simulink model "TASARIM"  (R2024a)
settings: Solver=VariableStepAuto  StartTime=0.0  StopTime=5  RelTol=1e-3
values from neighbouring files (symbols this model uses):
  B = 0.02    [PID_projesi_son_hal.m]
  dz = cell2mat(dz)    [PID_projesi_son_hal.m]
  j = 0.072    [PID_projesi_son_hal.m]
  K_i = 1.24    [PID_projesi_son_hal.m]
  Kb = 1.24    [PID_projesi_son_hal.m]
  Kd = (z1/sin(beta))*(((Ki*sin(beta))/(z1-2*cos(beta)+(1/z1)))+(sin(fi)/Gp_z1))    [PID_projesi_son_hal.m]
  Ki = Kv*T/limit    [PID_projesi_son_hal.m]
  Kp = (-cos(fi)/Gp_z1)-(2*Ki*z1*((z1-cos(beta))/(z1^2-2*z1*cos(beta)+1)))+((-z1*sin(fi)+cos(beta)*sin(fi))/(Gp_z1*sin(beta)))    [PID_projesi_son_hal.m]
  La = 1.4    [PID_projesi_son_hal.m]
  nz = cell2mat(nz)    [PID_projesi_son_hal.m]
  R = 2.8    [PID_projesi_son_hal.m]
  Ref = 24    [PID_projesi_son_hal.m]
  Ref_max = 24    [PID_projesi_son_hal.m]
  Ref_min = 24    [PID_projesi_son_hal.m]
  T = 10e-3    (= 0.01)    [PID_projesi_son_hal.m]
  Ts = T    [PID_projesi_son_hal.m]
libraries: spsIGBTDiodeLib x16, simulink_extras x11, simulink x8, spsDCMachineLib x4, spsDCVoltageSourceLib x4, spsGroundLib x4, spsVoltageMeasurementLib x4, sps_lib x1
settings Model: Creator=ESMA  LastModifiedBy=ESMA

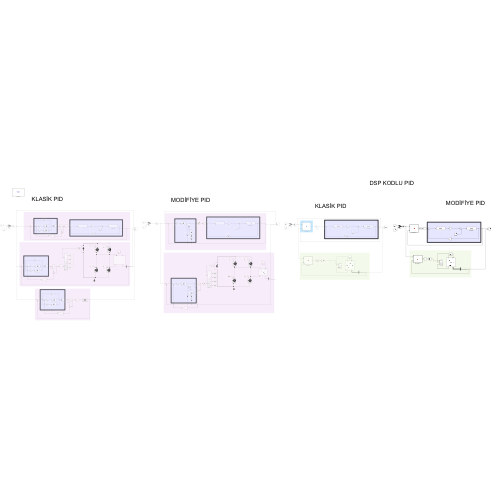
[thumbnail: Simulink's stored preview of the top-level diagram]
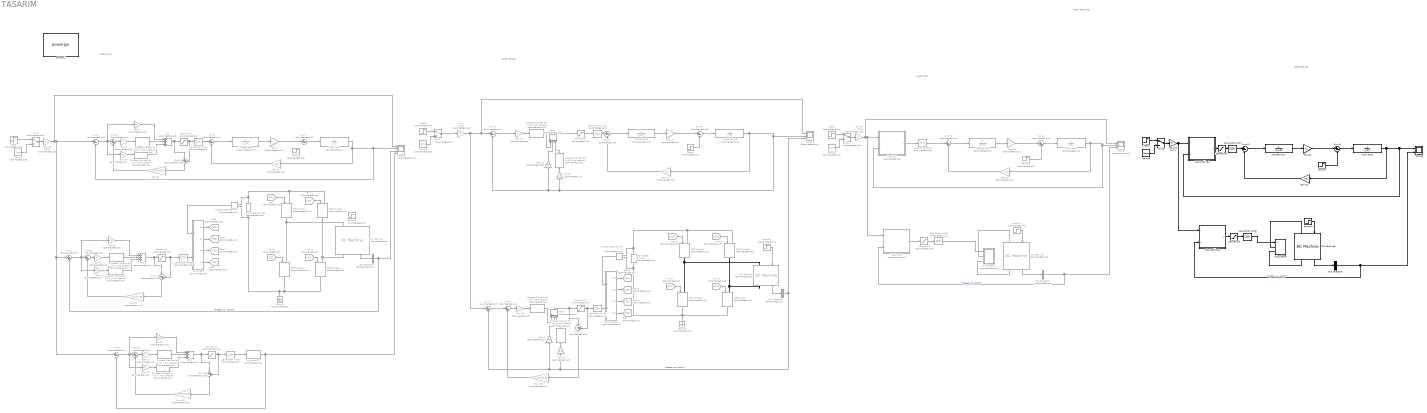
== system TASARIM ==
  note: KLASİK PID
  note: KLASİK PID
  note: MODİFİYE PID
  note: DSP KODLU PID
  note: MODİFİYE PID
  Add : Sum  Commented=on  Inputs=+++
  Add1 : Sum  Commented=on  Inputs=+--
  Add2 : Sum  Commented=on  Inputs=+++
  Add3 : Sum  Commented=on  Inputs=+--
  Add4 : Sum  Commented=on  Inputs=+++
  Bus Selector1 : BusSelector  Commented=on  OutputSignals=Speed wm (rad/s)
  Bus Selector2 : BusSelector  Commented=on  OutputSignals=Speed wm (rad/s)
  Bus Selector3 : BusSelector  OutputSignals=Speed wm (rad/s)
  Bus Selector4 : BusSelector  Commented=on  OutputSignals=Speed wm (rad/s)
  DC Machine : spsDCMachineLib/DC Machine  Commented=on  PresetModel=No  MechanicalLoad=Torque TL  FieldType=Permanent magnet  ShowDetailedParameters=on  MeasurementBus=off  RLa=[R La ]  RLf="[ 240  120]"  Laf=1.8  MachineConstant=Back-emf constant (V/rpm)  Ke=Kb*(2*pi)/60  Kt=1.8  J=j  Bm=B  Tf=0  w0=0  Ifinit=1  TsPowergui=0  TsBlock=-1
  DC Machine1 : spsDCMachineLib/DC Machine  Commented=on  PresetModel=No  MechanicalLoad=Torque TL  FieldType=Permanent magnet  ShowDetailedParameters=on  MeasurementBus=off  RLa=[R La ]  RLf="[ 240  120]"  Laf=1.8  MachineConstant=Back-emf constant (V/rpm)  Ke=Kb*(2*pi)/60  Kt=1.8  J=j  Bm=B  Tf=0  w0=0  Ifinit=1  TsPowergui=0  TsBlock=-1
  DC Machine2 : spsDCMachineLib/DC Machine  Commented=on  PresetModel=No  MechanicalLoad=Torque TL  FieldType=Permanent magnet  ShowDetailedParameters=on  MeasurementBus=off  RLa=[R La ]  RLf="[ 240  120]"  Laf=1.8  MachineConstant=Back-emf constant (V/rpm)  Ke=Kb*(2*pi)/60  Kt=1.8  J=j  Bm=B  Tf=0  w0=0  Ifinit=1  TsPowergui=0  TsBlock=-1
  DC Machine3 : spsDCMachineLib/DC Machine  PresetModel=No  MechanicalLoad=Torque TL  FieldType=Permanent magnet  ShowDetailedParameters=on  MeasurementBus=off  RLa=[R La ]  RLf="[ 240  120]"  Laf=1.8  MachineConstant=Back-emf constant (V/rpm)  Ke=Kb*(2*pi)/60  Kt=1.8  J=j  Bm=B  Tf=0  w0=0  Ifinit=1  TsPowergui=0  TsBlock=-1
  DC Voltage Source : spsDCVoltageSourceLib/DC Voltage Source  Commented=on  Amplitude=24  Measurements=None
  DC Voltage Source1 : spsDCVoltageSourceLib/DC Voltage Source  Commented=on  Amplitude=24  Measurements=None
  Discrete Transfer Fcn (with initial states){1..2,5,7,9} (5 alike) : simulink_extras/Additional Discrete/Discrete Transfer Fcn (with initial states)  Commented=on  N=[1 0]  D=[1 -1]  X0=[1]  TS=T
  Discrete Transfer Fcn (with initial states){3..4,6,8,10} (5 alike) : simulink_extras/Additional Discrete/Discrete Transfer Fcn (with initial states)  Commented=on  N=[1 -1]  D=[1 0]  X0=[1]  TS=T
  From : From  Commented=on  GotoTag=G1
  From1 : From  Commented=on  GotoTag=G3
  From2 : From  Commented=on  GotoTag=G4
  From3 : From  Commented=on  GotoTag=G2
  From4 : From  Commented=on  GotoTag=G11
  From5 : From  Commented=on  GotoTag=G31
  From6 : From  Commented=on  GotoTag=G41
  From7 : From  Commented=on  GotoTag=G21
  Gain{1,6,10,16..17} (5 alike) : Gain  Commented=on  Gain=Kd
  Gain11 : Gain  Commented=on  Gain=K_i
  Gain12 : Gain  Commented=on  Gain=Kb
  Gain{4,7..8,13,27} (5 alike) : Gain  Commented=on  Gain=Kp
  Gain{5,9,14..15,33} (5 alike) : Gain  Commented=on  Gain=Ki
  Gain{18,26,31..32} (4 alike) : Gain  Commented=on  Gain=Ki/Kd*4.35
  Gain19 : Gain  Commented=on  Gain=K_i
  Gain2 : Gain  Commented=on  Gain=K_i
  Gain20 : Gain  Commented=on  Gain=Kb
  Gain21 : Gain  Gain=K_i
  Gain22 : Gain  Gain=Kb
  Gain24 : Gain  Commented=on  Gain=18/24
  Gain25 : Gain  Gain=18/24
  Gain28 : Gain  Commented=on  Gain=18/24
  Gain3 : Gain  Commented=on  Gain=Kb
  Giriş : ManualSwitch  Commented=on
  Giriş1 : ManualSwitch  Commented=on
  Giriş2 : ManualSwitch  Commented=on
  Giriş3 : ManualSwitch
  Goto : Goto  Commented=on  GotoTag=G1
  Goto1 : Goto  Commented=on  GotoTag=G2
  Goto2 : Goto  Commented=on  GotoTag=G3
  Goto3 : Goto  Commented=on  GotoTag=G4
  Goto4 : Goto  Commented=on  GotoTag=G11
  Goto5 : Goto  Commented=on  GotoTag=G21
  Goto6 : Goto  Commented=on  GotoTag=G31
  Goto7 : Goto  Commented=on  GotoTag=G41
  Ground : spsGroundLib/Ground  Commented=on  LConnTagsString=a
  Ground1 : spsGroundLib/Ground  Commented=on  LConnTagsString=a
  IGBT/Diode{,1..7} (8 alike) : spsIGBTDiodeLib/IGBT//Diode  Commented=on  Ron=1e-6  Rs=1e5  Cs=inf  Measurements=off
  Klasik PID : MATLAB Function  Commented=on  TreatAsAtomicUnit=on
  Klasik PID1 : MATLAB Function  Commented=on  TreatAsAtomicUnit=on
  PID_Modifiye1 : MATLAB Function  TreatAsAtomicUnit=on
  PID_Modifiye2 : MATLAB Function  TreatAsAtomicUnit=on
  Ramp1 : simulink/Sources/Ramp  Commented=on  slope=Ref  start=0  InitialOutput=0
  Ramp2 : simulink/Sources/Ramp  Commented=on  slope=Ref  start=0  InitialOutput=0
  Ramp3 : simulink/Sources/Ramp  slope=Ref  start=0  InitialOutput=0
  Ramp4 : simulink/Sources/Ramp  Commented=on  slope=Ref  start=0  InitialOutput=0
  Saturation{1,3..4,7..9} (6 alike) : Saturate  Commented=on  UpperLimit=Ref  LowerLimit=-Ref
  Saturation5 : Saturate  UpperLimit=Ref  LowerLimit=-Ref
  Saturation6 : Saturate  UpperLimit=Ref  LowerLimit=-Ref
  Scope : Scope  Commented=on  NumInputPorts=3
  Scope1 : Scope  NumInputPorts=2
  Scope3 : Scope  Commented=on  NumInputPorts=3
  Scope4 : Scope  Commented=on  NumInputPorts=4
  Step1 : Step  Commented=on  Time=0  After=Ref  SampleTime=0
  Step2 : Step  Commented=on  Time=0  After=Ref  SampleTime=0
  Step3 : Step  Commented=on  Time=0  After=Ref  SampleTime=0
  Step4 : Step  Time=0  After=Ref  SampleTime=0
  Step5 : Step  Commented=on  Time=0  After=0  SampleTime=0
  Subsystem : Subsystem  Commented=on
  Subsystem1 : Subsystem  Commented=on
  Subsystem2 : Subsystem
  Subsystem3 : Subsystem  Commented=on
  Sum{1..5,7..9,11,13..14} (11 alike) : Sum  Commented=on  Inputs=|+-
  Sum{12,17,19,21} (4 alike) : Sum  Commented=on  Inputs=|-+
  Sum15 : Sum  Inputs=|+-
  Sum16 : Sum  Inputs=|+-
  Sum{6,18,20,22} (4 alike) : Sum  Commented=on  Inputs=|++
  Transfer Fcn1 : TransferFcn  Commented=on  Denominator=[La R]
  Transfer Fcn2 : TransferFcn  Denominator=[La R]
  Transfer Fcn3 : TransferFcn  Commented=on  Denominator=[La R]
  Transfer Fcn6 : TransferFcn  Commented=on  Denominator=[La R]
  Voltage Measurement : spsVoltageMeasurementLib/Voltage Measurement  Commented=on  PhasorSimulation=off  OutputType=Complex  PSBequivalent=0
  Voltage Measurement1 : spsVoltageMeasurementLib/Voltage Measurement  Commented=on  PhasorSimulation=off  OutputType=Complex  PSBequivalent=0
  Zero-Order Hold{1..6,9} (7 alike) : ZeroOrderHold  Commented=on  SampleTime=T
  Zero-Order Hold7 : ZeroOrderHold  SampleTime=T
  Zero-Order Hold8 : ZeroOrderHold  SampleTime=T
  bozucu{,1..3,5} (5 alike) : Step  Commented=on  Time=0  After=0  SampleTime=0
  bozucu4 : Step  Time=0  After=0  SampleTime=0
  bozucu6 : Step  Time=0  After=0  SampleTime=0
  giriş : Gain  Commented=on  Gain=18/24
  klasik PID : TransferFcn  Commented=on  Denominator=[j B]
  klasik PID1 : TransferFcn  Commented=on  Denominator=[j B]
  klasik PID2 : TransferFcn  Denominator=[j B]
  modifiyeli PID : TransferFcn  Commented=on  Denominator=[j B]
  powergui : sps_lib/powergui  Priority=1  SimulationMode=Discrete  SampleTime=1e-6  frequency=60  Iterations=50  frequencyindice=0  Pbase=100e6  ErrMax=1e-4  UnitsV=kV  UnitsW=MW  buscounter=0  FunctionMessages=off  echomessages=off  EnableUseOfTLC=off  CurrentSourceSwitches=off  DisableSnubberDevices=off  DisableRonSwitches=off  DisableVfSwitches=off  DisplayEquations=off  AutomaticDiscreteSolvers=off  SolverType=Tustin/Backward Euler (TBE)  Interpol=off  ExternalGateDelay=off  methode=off  Ts=100  x0status=blocks  SPID=on  SwTol=0  HookPort=off  NonlinearTolerance=1e-4  nMaxIteration=100  ContinueOnMaxIteration=off  RestoreLinks=warning  ResistiveCurrentMeasurement=off  Frange=[0:2:500]  Ylog=off  Xlog=on  ShowGrid=off  save=off  variable=ZData  structure=0  ZoomFFT=off  StartTime=0.0  cycles=1  DisplayStyle=1  fundamental=60  FreqAxis=off  MaxFrequency=1000  frequencyindicesteady=1  RmsSteady=1  display=off
  z_domeniTF : simulink_extras/Additional Discrete/Discrete Transfer Fcn (with initial states)  Commented=on  N=[nz]  D=[dz]  X0=[0]  TS=T
  wires:
  klasik PID/1 -> Gain3/1, Scope4/2, Sum2/2
  Gain7/1 -> Add/1
  Gain9/1 -> Discrete Transfer Fcn (with initial states)2/1
  Step2/1 -> Giriş/1
  Sum3/1 -> Transfer Fcn6/1
  Discrete Transfer Fcn (with initial states)3/1 -> Add/3
  Sum2/1 -> Gain7/1, Gain10/1, Sum20/1
  Sum7/1 -> klasik PID/1
  Gain10/1 -> Discrete Transfer Fcn (with initial states)3/1
  Transfer Fcn6/1 -> Gain2/1
  Ramp1/1 -> Giriş/2
  Gain2/1 -> Sum7/1
  Discrete Transfer Fcn (with initial states)2/1 -> Add/2
  Gain3/1 -> Sum3/2
  Discrete Transfer Fcn (with initial states)5/1 -> Add2/2
  Gain1/1 -> Discrete Transfer Fcn (with initial states)6/1
  Discrete Transfer Fcn (with initial states)6/1 -> Add2/3
  Gain4/1 -> Add2/1
  Gain5/1 -> Discrete Transfer Fcn (with initial states)5/1
  Sum1/1 -> Sum18/1, Gain1/1, Gain4/1
  Zero-Order Hold1/1 -> Sum3/1
  Sum11/1 -> modifiyeli PID/1
  Zero-Order Hold6/1 -> Subsystem3/1(uconT)
  bozucu5/1 -> DC Machine2/1
  DC Machine2/1 -> Bus Selector2/1
  Saturation1/1 -> Zero-Order Hold5/1, Sum12/2
  PID_Modifiye2/1(u) -> Saturation6/1
  Zero-Order Hold8/1 -> Subsystem2/1(uconT)
  Ramp2/1 -> Giriş2/2
  Gain8/1 -> Add3/2
  Gain22/1 -> Sum15/2
  Saturation6/1 -> Zero-Order Hold8/1
  Gain16/1 -> Discrete Transfer Fcn (with initial states)8/1
  bozucu2/1 -> DC Machine1/1
  Gain11/1 -> Sum11/1
  Subsystem1/1(G1) -> Goto4/1
  Gain15/1 -> Discrete Transfer Fcn (with initial states)7/1
  Step5/1 -> Sum11/2
  Zero-Order Hold5/1 -> Subsystem1/2(uconT)
  bozucu3/1 -> Sum14/2
  Zero-Order Hold4/1 -> Sum13/1
  Subsystem1/2(G2) -> Goto5/1
  Transfer Fcn1/1 -> Gain19/1
  Sum12/1 -> Gain18/1
  Subsystem1/4(G4) -> Goto7/1
  Gain14/1 -> Discrete Transfer Fcn (with initial states)1/1
  Sum4/1 -> Sum6/1
  Discrete Transfer Fcn (with initial states)8/1 -> Add3/3
  Gain25/1 -> PID_Modifiye2/1(r), PID_Modifiye1/1(r)
  Discrete Transfer Fcn (with initial states)1/1 -> Add1/1
  Ramp3/1 -> Giriş3/2
  PID_Modifiye1/1(u) -> Saturation5/1
  Transfer Fcn3/1 -> Gain11/1
  Discrete Transfer Fcn (with initial states)7/1 -> Add3/1
  Saturation3/1 -> Zero-Order Hold6/1
  Gain19/1 -> Sum14/1
  Sum16/1 -> klasik PID2/1
  Sum15/1 -> Transfer Fcn2/1
  Discrete Transfer Fcn (with initial states)4/1 -> Add1/3
  DC Machine1/1 -> Bus Selector1/1
  Gain6/1 -> Discrete Transfer Fcn (with initial states)4/1
  klasik PID2/1 -> Scope1/1, PID_Modifiye1/2(c), Gain22/1
  From5/1 -> IGBT/Diode5/1
  Zero-Order Hold2/1 -> Sum9/1
  Gain21/1 -> Sum16/1
  Zero-Order Hold7/1 -> Sum15/1
  Sum9/1 -> Transfer Fcn3/1
  Sum13/1 -> Transfer Fcn1/1
  Saturation5/1 -> Zero-Order Hold7/1
  Giriş1/1 -> giriş/1
  bozucu4/1 -> Sum16/2
  Step4/1 -> Giriş3/1
  Gain20/1 -> Sum13/2
  DC Machine3/1 -> Bus Selector3/1
  Transfer Fcn2/1 -> Gain21/1
  Gain18/1 -> Sum6/2
  Gain12/1 -> Sum9/2
  Subsystem1/3(G3) -> Goto6/1
  klasik PID1/1 -> Gain20/1, Scope/2, Klasik PID/2(c)
  Klasik PID1/1(u) -> Saturation3/1
  From6/1 -> IGBT/Diode7/1
  Step3/1 -> Giriş1/1
  From7/1 -> IGBT/Diode6/1
  From4/1 -> IGBT/Diode4/1
  Ramp4/1 -> Giriş1/2
  Step1/1 -> Giriş2/1
  Sum14/1 -> klasik PID1/1
  Gain13/1 -> Add1/2
  Klasik PID/1(u) -> Zero-Order Hold4/1
  Add1/1 -> Saturation4/1
  modifiyeli PID/1 -> Gain12/1, Gain6/1, Sum8/2, Gain13/1, Scope3/2
  Add3/1 -> Sum12/1, Saturation1/1
  Voltage Measurement1/1 -> Subsystem1/1(E)
  Sum8/1 -> Gain14/1
  Giriş2/1 -> Gain24/1
  bozucu6/1 -> DC Machine3/1
  Giriş3/1 -> Gain25/1
  giriş/1 -> Scope3/1, Sum8/1, Sum4/1
  Zero-Order Hold3/1 -> Subsystem/2(uconT)
  Voltage Measurement/1 -> Subsystem/1(E)
  From3/1 -> IGBT/Diode2/1
  Subsystem/1(G1) -> Goto/1
  From/1 -> IGBT/Diode/1
  Subsystem/2(G2) -> Goto1/1
  Subsystem/3(G3) -> Goto2/1
  From2/1 -> IGBT/Diode3/1
  DC Machine/1 -> Bus Selector4/1
  From1/1 -> IGBT/Diode1/1
  Subsystem/4(G4) -> Goto3/1
  Saturation4/1 -> Zero-Order Hold2/1
  z_domeniTF/1 -> Scope4/4, Sum5/2
  Add2/1 -> Saturation8/1, Sum17/1
  Gain31/1 -> Sum18/2
  Sum17/1 -> Gain31/1
  Sum18/1 -> Gain5/1
  Sum19/1 -> Gain32/1
  Add/1 -> Saturation7/1, Sum19/1
  Gain32/1 -> Sum20/2
  Sum20/1 -> Gain9/1
  Add4/1 -> Sum21/1, Saturation9/1
  Sum22/1 -> Gain33/1
  Sum5/1 -> Sum22/1, Gain17/1, Gain27/1
  Gain33/1 -> Discrete Transfer Fcn (with initial states)9/1
  Gain17/1 -> Discrete Transfer Fcn (with initial states)10/1
  Discrete Transfer Fcn (with initial states)9/1 -> Add4/2
  Discrete Transfer Fcn (with initial states)10/1 -> Add4/3
  Sum21/1 -> Gain26/1
  Gain26/1 -> Sum22/2
  Saturation9/1 -> Zero-Order Hold9/1, Sum21/2
  Gain27/1 -> Add4/1
  Zero-Order Hold9/1 -> z_domeniTF/1
  Bus Selector4/1 -> Scope4/3, Sum1/2  "<Speed wm (rad/s)>"
  Bus Selector1/1 -> Scope3/3, Gain16/1, Gain8/1, Sum4/2  "<Speed wm (rad/s)>"
  Sum6/1 -> Gain15/1
  Bus Selector3/1 -> Scope1/2, PID_Modifiye2/2(c)  "<Speed wm (rad/s)>"
  Bus Selector2/1 -> Scope/3, Klasik PID1/2(c)  "<Speed wm (rad/s)>"
  Saturation7/1 -> Sum19/2, Zero-Order Hold1/1
  Saturation8/1 -> Zero-Order Hold3/1, Sum17/2
  Giriş/1 -> Gain28/1
  Gain28/1 -> Scope4/1, Sum2/1, Sum1/1, Sum5/1
  Gain24/1 -> Scope/1, Klasik PID1/1(r), Klasik PID/1(r)
  connections:
  DC Machine1/RConn1 -- IGBT/Diode7/LConn1 -- IGBT/Diode5/RConn1
  Subsystem3/LConn1 -- DC Machine2/LConn1
  Subsystem3/LConn2 -- DC Machine2/RConn1
  Subsystem2/LConn1 -- DC Machine3/LConn1
  Subsystem2/LConn2 -- DC Machine3/RConn1
  Voltage Measurement1/LConn2 -- DC Voltage Source1/LConn1 -- IGBT/Diode7/RConn1 -- IGBT/Diode6/RConn1 -- Ground1/LConn1
  DC Voltage Source1/RConn1 -- Voltage Measurement1/LConn1 -- IGBT/Diode5/LConn1 -- IGBT/Diode4/LConn1
  DC Machine1/LConn1 -- IGBT/Diode4/RConn1 -- IGBT/Diode6/LConn1
  DC Machine/RConn1 -- IGBT/Diode3/LConn1 -- IGBT/Diode1/RConn1
  DC Voltage Source/RConn1 -- Voltage Measurement/LConn1 -- IGBT/Diode1/LConn1 -- IGBT/Diode/LConn1
  DC Machine/LConn1 -- IGBT/Diode2/LConn1 -- IGBT/Diode/RConn1
  Voltage Measurement/LConn2 -- DC Voltage Source/LConn1 -- Ground/LConn1 -- IGBT/Diode2/RConn1 -- IGBT/Diode3/RConn1

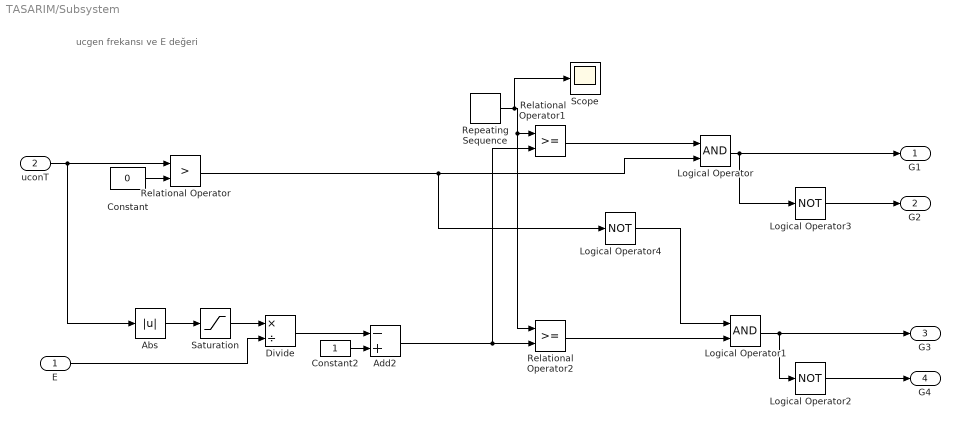
== system TASARIM/Subsystem ==
  note: ucgen frekansı ve E değeri
  E : Inport
  uconT : Inport  Port=2
  Abs : Abs  SaturateOnIntegerOverflow=off
  Add2 : Sum  Inputs=-+
  Constant : Constant  Value=0
  Constant2 : Constant
  Divide : Product  Inputs=*/
  Logical Operator : Logic  AllPortsSameDT=off  OutDataTypeStr=boolean
  Logical Operator1 : Logic  AllPortsSameDT=off  OutDataTypeStr=boolean
  Logical Operator2 : Logic  Operator=NOT  AllPortsSameDT=off  OutDataTypeStr=boolean
  Logical Operator3 : Logic  Operator=NOT  AllPortsSameDT=off  OutDataTypeStr=boolean
  Logical Operator4 : Logic  Operator=NOT  AllPortsSameDT=off  OutDataTypeStr=boolean
  Relational Operator : RelationalOperator  Operator=>  OutDataTypeStr=boolean  RndMeth=Simplest  InputSameDT=off
  Relational Operator1 : RelationalOperator  OutDataTypeStr=boolean  RndMeth=Simplest  InputSameDT=off
  Relational Operator2 : RelationalOperator  OutDataTypeStr=boolean  RndMeth=Simplest  InputSameDT=off
  Repeating Sequence : simulink/Sources/Repeating Sequence  rep_seq_t=[0 0.5 1]*T  rep_seq_y="[0 1  0]"
  Saturation : Saturate  UpperLimit=24
  Scope : Scope
  G1 : Outport
  G2 : Outport  Port=2
  G3 : Outport  Port=3
  G4 : Outport  Port=4
  wires:
  Constant/1 -> Relational Operator/2
  E/1 -> Divide/2
  Logical Operator3/1 -> G2/1
  Abs/1 -> Saturation/1
  Relational Operator2/1 -> Logical Operator1/2
  Relational Operator/1 -> Logical Operator4/1, Logical Operator/2
  uconT/1 -> Relational Operator/1, Abs/1
  Saturation/1 -> Divide/1
  Logical Operator/1 -> G1/1, Logical Operator3/1
  Relational Operator1/1 -> Logical Operator/1
  Logical Operator1/1 -> Logical Operator2/1, G3/1
  Divide/1 -> Add2/1
  Logical Operator4/1 -> Logical Operator1/1
  Constant2/1 -> Add2/2
  Logical Operator2/1 -> G4/1
  Add2/1 -> Relational Operator1/2, Relational Operator2/2
  Repeating Sequence/1 -> Scope/1, Relational Operator2/1, Relational Operator1/1

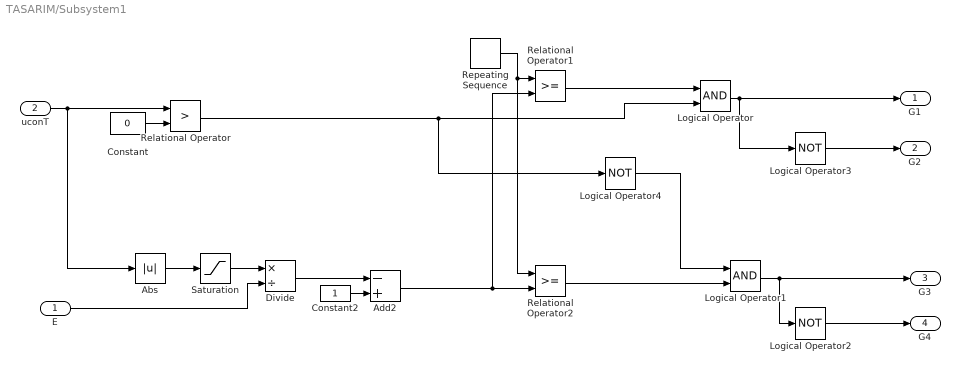
== system TASARIM/Subsystem1 ==
  E : Inport
  uconT : Inport  Port=2
  Abs : Abs  SaturateOnIntegerOverflow=off
  Add2 : Sum  Inputs=-+
  Constant : Constant  Value=0
  Constant2 : Constant
  Divide : Product  Inputs=*/
  Logical Operator : Logic  AllPortsSameDT=off  OutDataTypeStr=boolean
  Logical Operator1 : Logic  AllPortsSameDT=off  OutDataTypeStr=boolean
  Logical Operator2 : Logic  Operator=NOT  AllPortsSameDT=off  OutDataTypeStr=boolean
  Logical Operator3 : Logic  Operator=NOT  AllPortsSameDT=off  OutDataTypeStr=boolean
  Logical Operator4 : Logic  Operator=NOT  AllPortsSameDT=off  OutDataTypeStr=boolean
  Relational Operator : RelationalOperator  Operator=>  OutDataTypeStr=boolean  RndMeth=Simplest  InputSameDT=off
  Relational Operator1 : RelationalOperator  OutDataTypeStr=boolean  RndMeth=Simplest  InputSameDT=off
  Relational Operator2 : RelationalOperator  OutDataTypeStr=boolean  RndMeth=Simplest  InputSameDT=off
  Repeating Sequence : simulink/Sources/Repeating Sequence  rep_seq_t=[0 1 2]*0.5*T  rep_seq_y=[0 1 0]
  Saturation : Saturate  UpperLimit=Ref  LowerLimit=-Ref
  G1 : Outport
  G2 : Outport  Port=2
  G3 : Outport  Port=3
  G4 : Outport  Port=4
  wires:
  Constant/1 -> Relational Operator/2
  E/1 -> Divide/2
  Logical Operator3/1 -> G2/1
  Abs/1 -> Saturation/1
  Relational Operator2/1 -> Logical Operator1/2
  Relational Operator/1 -> Logical Operator4/1, Logical Operator/2
  uconT/1 -> Relational Operator/1, Abs/1
  Saturation/1 -> Divide/1
  Logical Operator/1 -> G1/1, Logical Operator3/1
  Relational Operator1/1 -> Logical Operator/1
  Logical Operator1/1 -> Logical Operator2/1, G3/1
  Divide/1 -> Add2/1
  Logical Operator4/1 -> Logical Operator1/1
  Constant2/1 -> Add2/2
  Logical Operator2/1 -> G4/1
  Add2/1 -> Relational Operator1/2, Relational Operator2/2
  Repeating Sequence/1 -> Relational Operator2/1, Relational Operator1/1

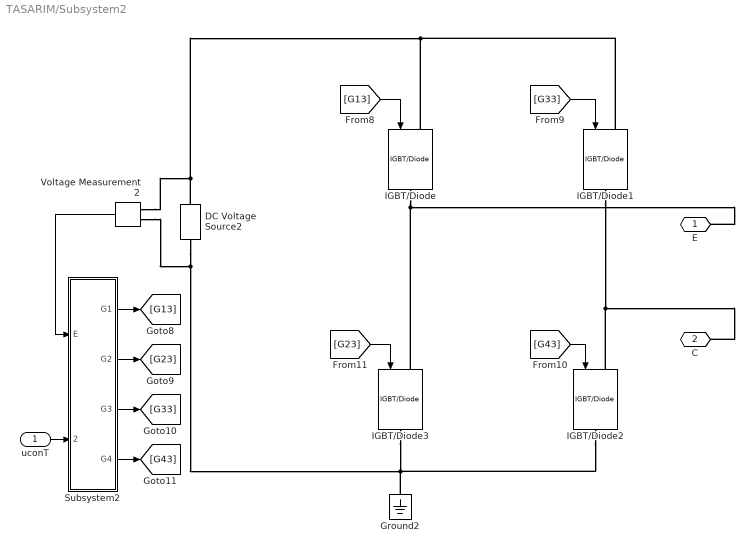
== system TASARIM/Subsystem2 ==
  uconT : Inport
  DC Voltage Source2 : spsDCVoltageSourceLib/DC Voltage Source  Amplitude=24  Measurements=None
  Ground2 : spsGroundLib/Ground  LConnTagsString=a
  IGBT/Diode{,1..3} (4 alike) : spsIGBTDiodeLib/IGBT//Diode  Ron=1e-6  Rs=1e5  Cs=inf  Measurements=off
  Subsystem2 : Subsystem
  Voltage Measurement2 : spsVoltageMeasurementLib/Voltage Measurement  PhasorSimulation=off  OutputType=Complex  PSBequivalent=0
  E : PMIOPort  Side=Left
  C : PMIOPort  Port=2  Side=Left
  wires:
  [G13] -> IGBT/Diode/1
  [G33] -> IGBT/Diode1/1
  [G43] -> IGBT/Diode2/1
  Subsystem2/3(G3) -> [G33]
  [G23] -> IGBT/Diode3/1
  Subsystem2/1(G1) -> [G13]
  Voltage Measurement2/1 -> Subsystem2/1(E)
  Subsystem2/4(G4) -> [G43]
  Subsystem2/2(G2) -> [G23]
  uconT/1 -> Subsystem2/2(uconT)
  connections:
  DC Voltage Source2/LConn1 -- IGBT/Diode3/RConn1 -- IGBT/Diode2/RConn1 -- Ground2/LConn1 -- Voltage Measurement2/LConn2
  Voltage Measurement2/LConn1 -- IGBT/Diode1/LConn1 -- IGBT/Diode/LConn1 -- DC Voltage Source2/RConn1
  C/RConn1 -- IGBT/Diode2/LConn1 -- IGBT/Diode1/RConn1
  E/RConn1 -- IGBT/Diode3/LConn1 -- IGBT/Diode/RConn1

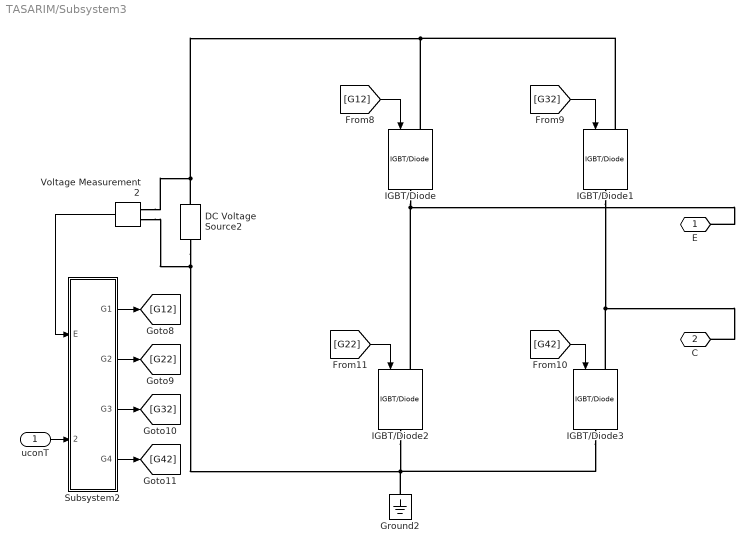
== system TASARIM/Subsystem3 ==
  uconT : Inport
  DC Voltage Source2 : spsDCVoltageSourceLib/DC Voltage Source  Amplitude=24  Measurements=None
  Ground2 : spsGroundLib/Ground  LConnTagsString=a
  IGBT/Diode{,1..3} (4 alike) : spsIGBTDiodeLib/IGBT//Diode  Ron=1e-6  Rs=1e5  Cs=inf  Measurements=off
  Subsystem2 : Subsystem
  Voltage Measurement2 : spsVoltageMeasurementLib/Voltage Measurement  PhasorSimulation=off  OutputType=Complex  PSBequivalent=0
  E : PMIOPort  Side=Left
  C : PMIOPort  Port=2  Side=Left
  wires:
  [G12] -> IGBT/Diode/1
  [G32] -> IGBT/Diode1/1
  [G42] -> IGBT/Diode3/1
  Subsystem2/3(G3) -> [G32]
  [G22] -> IGBT/Diode2/1
  Subsystem2/1(G1) -> [G12]
  Voltage Measurement2/1 -> Subsystem2/1(E)
  Subsystem2/4(G4) -> [G42]
  Subsystem2/2(G2) -> [G22]
  uconT/1 -> Subsystem2/2(uconT)
  connections:
  DC Voltage Source2/LConn1 -- IGBT/Diode3/RConn1 -- IGBT/Diode2/RConn1 -- Ground2/LConn1 -- Voltage Measurement2/LConn2
  Voltage Measurement2/LConn1 -- IGBT/Diode1/LConn1 -- IGBT/Diode/LConn1 -- DC Voltage Source2/RConn1
  C/RConn1 -- IGBT/Diode3/LConn1 -- IGBT/Diode1/RConn1
  E/RConn1 -- IGBT/Diode2/LConn1 -- IGBT/Diode/RConn1

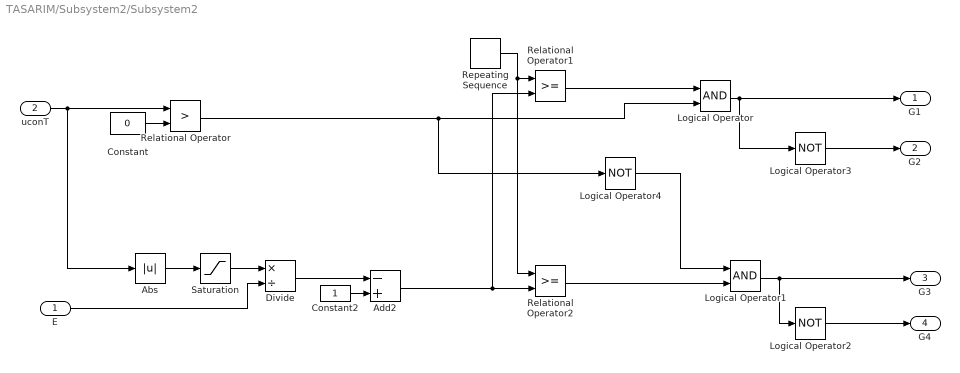
== system TASARIM/Subsystem2/Subsystem2 ==
  E : Inport
  uconT : Inport  Port=2
  Abs : Abs  SaturateOnIntegerOverflow=off
  Add2 : Sum  Inputs=-+
  Constant : Constant  Value=0
  Constant2 : Constant
  Divide : Product  Inputs=*/
  Logical Operator : Logic  AllPortsSameDT=off  OutDataTypeStr=boolean
  Logical Operator1 : Logic  AllPortsSameDT=off  OutDataTypeStr=boolean
  Logical Operator2 : Logic  Operator=NOT  AllPortsSameDT=off  OutDataTypeStr=boolean
  Logical Operator3 : Logic  Operator=NOT  AllPortsSameDT=off  OutDataTypeStr=boolean
  Logical Operator4 : Logic  Operator=NOT  AllPortsSameDT=off  OutDataTypeStr=boolean
  Relational Operator : RelationalOperator  Operator=>  OutDataTypeStr=boolean  RndMeth=Simplest  InputSameDT=off
  Relational Operator1 : RelationalOperator  OutDataTypeStr=boolean  RndMeth=Simplest  InputSameDT=off
  Relational Operator2 : RelationalOperator  OutDataTypeStr=boolean  RndMeth=Simplest  InputSameDT=off
  Repeating Sequence : simulink/Sources/Repeating Sequence  rep_seq_t=[0 1 2]*0.5*T  rep_seq_y=[0 1 0]
  Saturation : Saturate  UpperLimit=Ref  LowerLimit=-Ref
  G1 : Outport
  G2 : Outport  Port=2
  G3 : Outport  Port=3
  G4 : Outport  Port=4
  wires:
  Constant/1 -> Relational Operator/2
  E/1 -> Divide/2
  Logical Operator3/1 -> G2/1
  Abs/1 -> Saturation/1
  Relational Operator2/1 -> Logical Operator1/2
  Relational Operator/1 -> Logical Operator4/1, Logical Operator/2
  uconT/1 -> Relational Operator/1, Abs/1
  Saturation/1 -> Divide/1
  Logical Operator/1 -> G1/1, Logical Operator3/1
  Relational Operator1/1 -> Logical Operator/1
  Logical Operator1/1 -> Logical Operator2/1, G3/1
  Divide/1 -> Add2/1
  Logical Operator4/1 -> Logical Operator1/1
  Constant2/1 -> Add2/2
  Logical Operator2/1 -> G4/1
  Add2/1 -> Relational Operator1/2, Relational Operator2/2
  Repeating Sequence/1 -> Relational Operator2/1, Relational Operator1/1

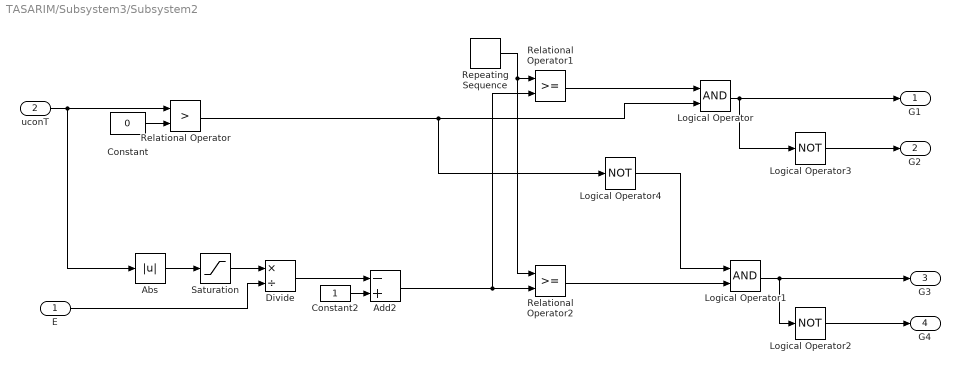
== system TASARIM/Subsystem3/Subsystem2 ==
  E : Inport
  uconT : Inport  Port=2
  Abs : Abs  SaturateOnIntegerOverflow=off
  Add2 : Sum  Inputs=-+
  Constant : Constant  Value=0
  Constant2 : Constant
  Divide : Product  Inputs=*/
  Logical Operator : Logic  AllPortsSameDT=off  OutDataTypeStr=boolean
  Logical Operator1 : Logic  AllPortsSameDT=off  OutDataTypeStr=boolean
  Logical Operator2 : Logic  Operator=NOT  AllPortsSameDT=off  OutDataTypeStr=boolean
  Logical Operator3 : Logic  Operator=NOT  AllPortsSameDT=off  OutDataTypeStr=boolean
  Logical Operator4 : Logic  Operator=NOT  AllPortsSameDT=off  OutDataTypeStr=boolean
  Relational Operator : RelationalOperator  Operator=>  OutDataTypeStr=boolean  RndMeth=Simplest  InputSameDT=off
  Relational Operator1 : RelationalOperator  OutDataTypeStr=boolean  RndMeth=Simplest  InputSameDT=off
  Relational Operator2 : RelationalOperator  OutDataTypeStr=boolean  RndMeth=Simplest  InputSameDT=off
  Repeating Sequence : simulink/Sources/Repeating Sequence  rep_seq_t=[0 1 2]*0.5*T  rep_seq_y=[0 1 0]
  Saturation : Saturate  UpperLimit=Ref  LowerLimit=-Ref
  G1 : Outport
  G2 : Outport  Port=2
  G3 : Outport  Port=3
  G4 : Outport  Port=4
  wires:
  Constant/1 -> Relational Operator/2
  E/1 -> Divide/2
  Logical Operator3/1 -> G2/1
  Abs/1 -> Saturation/1
  Relational Operator2/1 -> Logical Operator1/2
  Relational Operator/1 -> Logical Operator4/1, Logical Operator/2
  uconT/1 -> Relational Operator/1, Abs/1
  Saturation/1 -> Divide/1
  Logical Operator/1 -> G1/1, Logical Operator3/1
  Relational Operator1/1 -> Logical Operator/1
  Logical Operator1/1 -> Logical Operator2/1, G3/1
  Divide/1 -> Add2/1
  Logical Operator4/1 -> Logical Operator1/1
  Constant2/1 -> Add2/2
  Logical Operator2/1 -> G4/1
  Add2/1 -> Relational Operator1/2, Relational Operator2/2
  Repeating Sequence/1 -> Relational Operator2/1, Relational Operator1/1

== matlab function TASARIM/PID_Modifiye1 ==
  settings: updateMethod=DISCRETE  sampleTime=Ts
  data: r input; u output; c input; Ki parameter; Kd parameter; Kp parameter; Ts parameter; Ref_min parameter; Ref_max parameter
function u = fcn(r, c, Ki, Kd, Kp, Ts, Ref_min, Ref_max)
    persistent A B;
    if isempty(A), A = 0; end
    if isempty(B), B = 0; end


    e = r - c; 
    up = Kp * c; 
    x = e + A;        
    ui = Ki * x;      
    A=x;   
    ud = Kd * (c - B);   
    B=c;
    
    u_raw = ui - up - ud;

    u = max(min(u_raw, Ref_max), Ref_min);
    if u == u_raw
        % Saturasyon yok
        A = x;
    else
        % Saturasyon var

    end

    B = c;

    pause(Ts);
end

== matlab function TASARIM/Klasik PID ==
  settings: updateMethod=DISCRETE  sampleTime=Ts
  data: r input; u output; c input; Ki parameter; Kd parameter; Kp parameter; Ts parameter; Ref_min parameter; Ref_max parameter
function u = fcn(r,c, Ki, Kd, Kp, Ts, Ref_min, Ref_max)
    persistent A B;

    if (isempty(A) && isempty(B))
        A = 0;
        B = 0;
    end

    e = r - c; 

    up = Kp * e;          
    x = e + A;           
    ui = Ki * x;          
    ud = Kd * (e - B);    

    u_raw = up + ui + ud;

    u = max(min(u_raw, Ref_max), Ref_min);

    if u == u_raw
        % Saturasyon yok
        A = x;
    else
        % Saturasyon var
        % Anti-windup etkisi
    end
    B = e; 

    pause(Ts);
end

== matlab function TASARIM/Klasik PID1 ==
  settings: updateMethod=DISCRETE  sampleTime=Ts
  data: r input; u output; c input; Ki parameter; Kd parameter; Kp parameter; Ts parameter; Ref_min parameter; Ref_max parameter
function u = fcn(r, c, Ki, Kd, Kp, Ts, Ref_min, Ref_max)
    persistent A B;

    if (isempty(A) && isempty(B))
        A = 0;
        B = 0;
    end

    e = r- c; 

    up = Kp * e;          
    x = e + A;           
    ui = Ki * x;          
    ud = Kd * (e - B);    

    u_raw = up + ui + ud;

    u = max(min(u_raw, Ref_max), Ref_min);

    if u == u_raw
        % Saturasyon yok
        A = x;
    else
        % Saturasyon var
        % Anti-windup etkisi
    end
    B = e; 

    pause(Ts);
end

== matlab function TASARIM/PID_Modifiye2 ==
  settings: updateMethod=DISCRETE  sampleTime=Ts
  data: r input; u output; c input; Ki parameter; Kd parameter; Kp parameter; Ts parameter; Ref_min parameter; Ref_max parameter
function u = fcn(r, c, Ki, Kd, Kp, Ts, Ref_min, Ref_max)
    persistent A B;
    if isempty(A), A = 0; end
    if isempty(B), B = 0; end


    e = r - c; 
    x = e + A;        
    ui = Ki * x;      
    up = Kp * c;      
    ud = Kd * (c - B);   

    u_raw = ui - up - ud;

    u = max(min(u_raw, Ref_max), Ref_min);
    if u == u_raw
        % Saturasyon yok
        A = x;
    else
        % Saturasyon var

    end

    B = c;

    pause(Ts);
end
